simulink library "pixhawk_slib_rfly"  (R2022b)
settings: Solver=ode45  StartTime=0.0  StopTime=10.0  RelTol=1e-3
libraries: pixhawk_slib_uORB_RW x42, $bdroot x7
(part 2 of 3)

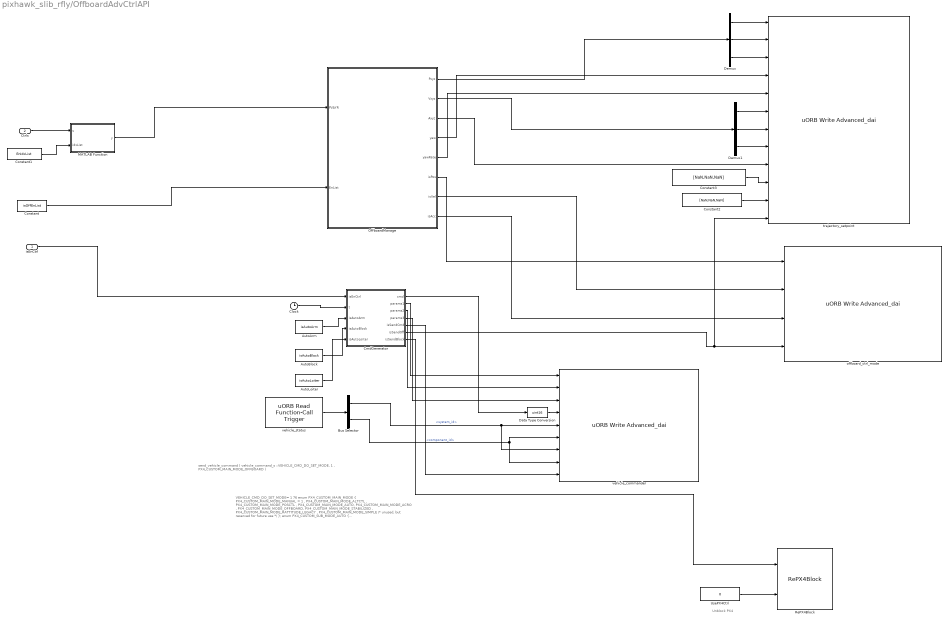
== system pixhawk_slib_rfly/OffboardAdvCtrlAPI ==
  note: VEHICLE_CMD_DO_SET_MODE= 1 76
      |
      | enum PX4_CUSTOM_MAIN_MODE {
      | PX4_CUSTOM_MAIN_MODE_MANUAL = 1 ,
      | PX4_CUSTOM_MAIN_MODE_ALTCTL ,
      | PX4_CUSTOM_MAIN_MODE_POSCTL ,
      | PX4_CUSTOM_MAIN_MODE_AUTO,
      | PX4_CUSTOM_MAIN_MODE_ACRO ,
      | PX4_CUSTOM_MAIN_MODE_OFFBOARD,
      | PX4_CUSTOM_MAIN_MODE_STABILIZED ,
      | PX4_CUSTOM_MAIN_MODE_RATTITUDE_LEGACY ,
      | PX4_CUSTOM_MAIN_MODE_SIMPLE /* unused, but reserved for future use */
      | };
      |
      | enum PX4_CUSTOM_SUB_MODE_AUTO {
      | PX4_CUSTOM_SUB_MODE_AUTO_READY = 1 ,
      | PX4_CUSTOM_SUB_MODE_AUTO_TAKEOFF ,
      | PX4_CUSTOM_SUB_MODE_AUTO_LOITER,
      | PX4_CUSTOM_SUB_MODE_AUTO_MISSION ,
      | PX4_CUSTOM_SUB_MODE_AUTO_RTL ,
      | PX4_CUSTOM_SUB_MODE_AUTO_LAND ,
      | PX4_CUSTOM_SUB_MODE_AUTO_RESERVED_DO_NOT_USE , // was PX4_CUSTOM_SUB_MODE_AUTO_RTGS, deleted 2020-03-05
      | PX4_CUSTOM_SUB_MODE_AUTO_FOLLOW_TARGET ,
      | PX4_CUSTOM_SUB_MODE_AUTO_PRECLAND
      | };
  note: Unblock PX4
  note: send_vehicle_command ( vehicle_command_s ::VEHICLE_CMD_DO_SET_MODE, 1 , PX4_CUSTOM_MAIN_MODE_OFFBOARD )
  isEnCtrl : Inport  OutDataTypeStr=boolean  PortDimensions=1
  Ctrls : Inport  Port=2  OutDataTypeStr=single  PortDimensions=4
  AutoArm : Constant  Value=isAutoArm  OutDataTypeStr=boolean
  AutoBlock : Constant  Value=isAutoBlock  OutDataTypeStr=boolean
  AutoLoiter : Constant  Value=isAutoLoiter  OutDataTypeStr=boolean
  Bus Selector : BusSelector  OutputSignals=system_id,component_id
  Clock : Clock
  CmdGenerator : MATLAB Function  TreatAsAtomicUnit=on  SystemSampleTime=SamTime
  Constant : Constant  Value=isOffEnList  OutDataTypeStr=boolean
  Constant1 : Constant  Value=EnIdxList
  Constant2 : Constant  Value=[NaN,NaN,NaN]  OutDataTypeStr=single
  Constant3 : Constant  Value=[NaN,NaN,NaN]  OutDataTypeStr=single
  Data Type Conversion : DataTypeConversion  OutDataTypeStr=uint16  SaturateOnIntegerOverflow=off  RndMeth=Floor
  Demux : Demux  Outputs=3
  Demux1 : Demux  Outputs=3
  MATLAB Function : MATLAB Function  TreatAsAtomicUnit=on  SystemSampleTime=SamTime
  OffboardManage : MATLAB Function  TreatAsAtomicUnit=on  SystemSampleTime=SamTime
  RePX4Block : $bdroot/RePX4Block  SamTime=SamTime
  UsePX4Ctrl : Constant  Value=0  OutDataTypeStr=uint8
  offboard_ctrl_mode : pixhawk_slib_uORB_RW/uORB Write Advanced_dai  Ts=0  uORB_AdvtQueue=on  uORB_FieldEnabledArr="0  0  0  1  0  0  0  0  0  0  0"  uORB_Topic_str=0  uORB_Topic_str_ID=0  uORB_Struct_DT="[1  1  1  1  1]"  BlockInputCount=5  uORB_StructParams="[\"voltage_v\",\"voltage_filtered_v\",\"current_a\",\"current_filtered_a\",\"remaining\"]"  uORB_PortSizes="[1  1  1  1]"  MsgSizeOf=0  MW_update=true
      settings: SourceProductName=Pixhawk Target Blocks
  trajectory_setpoint : pixhawk_slib_uORB_RW/uORB Write Advanced_dai  Ts=0  uORB_AdvtQueue=on  uORB_FieldEnabledArr="0  0  0  1  0  0  0  0  0  0  0"  uORB_Topic_str=0  uORB_Topic_str_ID=0  uORB_Struct_DT="[1  1  1  1  1]"  BlockInputCount=5  uORB_StructParams="[\"voltage_v\",\"voltage_filtered_v\",\"current_a\",\"current_filtered_a\",\"remaining\"]"  uORB_PortSizes="[1  1  1  1]"  MsgSizeOf=0  MW_update=true
      settings: SourceProductName=Pixhawk Target Blocks
  vehicle_commander : pixhawk_slib_uORB_RW/uORB Write Advanced_dai  Ts=0  uORB_AdvtQueue=on  uORB_FieldEnabledArr="0  0  0  1  0  0  0  0  0  0  0"  uORB_Topic_str=0  uORB_Topic_str_ID=0  uORB_Struct_DT="[1  1  1  1  1]"  BlockInputCount=5  uORB_StructParams="[\"voltage_v\",\"voltage_filtered_v\",\"current_a\",\"current_filtered_a\",\"remaining\"]"  uORB_PortSizes="[1  1  1  1]"  MsgSizeOf=0  MW_update=true
      settings: SourceProductName=Pixhawk Target Blocks
  vehicle_status : pixhawk_slib_uORB_RW/uORB Read Function-Call Trigger  uORB_Topic_str='vehicle_status'  BusObjVar=Bus: vehicle_status_SL  uORB_Interval=50  AsyncOutput=off  Fcn_call_select=Generate Function Call Signal  TaskName='Task1'  Poll_timeout=-1  Ts=SamTime
      settings: SourceProductName=Pixhawk Target Blocks
  wires:
  Ctrls/1 -> MATLAB Function/1(u)
  Constant1/1 -> MATLAB Function/2(idxList)
  Bus Selector/2 -> vehicle_commander/8, vehicle_commander/6  "<component_id>"
  CmdGenerator/5(isSendCmd) -> vehicle_commander/9
  Clock/1 -> CmdGenerator/2(t)
  OffboardManage/6(isPos) -> offboard_ctrl_mode/1
  OffboardManage/7(isVel) -> offboard_ctrl_mode/2
  AutoLoiter/1 -> CmdGenerator/5(isAutoLoiter)
  UsePX4Ctrl/1 -> RePX4Block/2
  AutoBlock/1 -> CmdGenerator/4(isAutoBlock)
  Constant/1 -> OffboardManage/2(EnList)
  CmdGenerator/4(params3) -> vehicle_commander/3
  CmdGenerator/1(cmd) -> Data Type Conversion/1
  CmdGenerator/3(params2) -> vehicle_commander/2
  AutoArm/1 -> CmdGenerator/3(isAutoArm)
  OffboardManage/8(isAcc) -> offboard_ctrl_mode/3
  CmdGenerator/2(params1) -> vehicle_commander/1
  CmdGenerator/7(isSendBlock) -> RePX4Block/1
  vehicle_status/1 -> Bus Selector/1
  MATLAB Function/1(y) -> OffboardManage/1(PVAYR)
  Bus Selector/1 -> vehicle_commander/7, vehicle_commander/5  "<system_id>"
  isEnCtrl/1 -> CmdGenerator/1(isEnCtrl)
  Demux1/3 -> trajectory_setpoint/8
  Demux1/1 -> trajectory_setpoint/6
  Demux/3 -> trajectory_setpoint/3
  Demux1/2 -> trajectory_setpoint/7
  Demux/1 -> trajectory_setpoint/1
  Demux/2 -> trajectory_setpoint/2
  OffboardManage/5(yawRate) -> trajectory_setpoint/5
  OffboardManage/3(Axyz) -> trajectory_setpoint/9
  Constant2/1 -> trajectory_setpoint/11
  OffboardManage/4(yaw) -> trajectory_setpoint/4
  Constant3/1 -> trajectory_setpoint/10
  OffboardManage/1(Pxyz) -> Demux/1
  CmdGenerator/6(isSendOff) -> trajectory_setpoint/12, offboard_ctrl_mode/4
  OffboardManage/2(Vxyz) -> Demux1/1
  Data Type Conversion/1 -> vehicle_commander/4

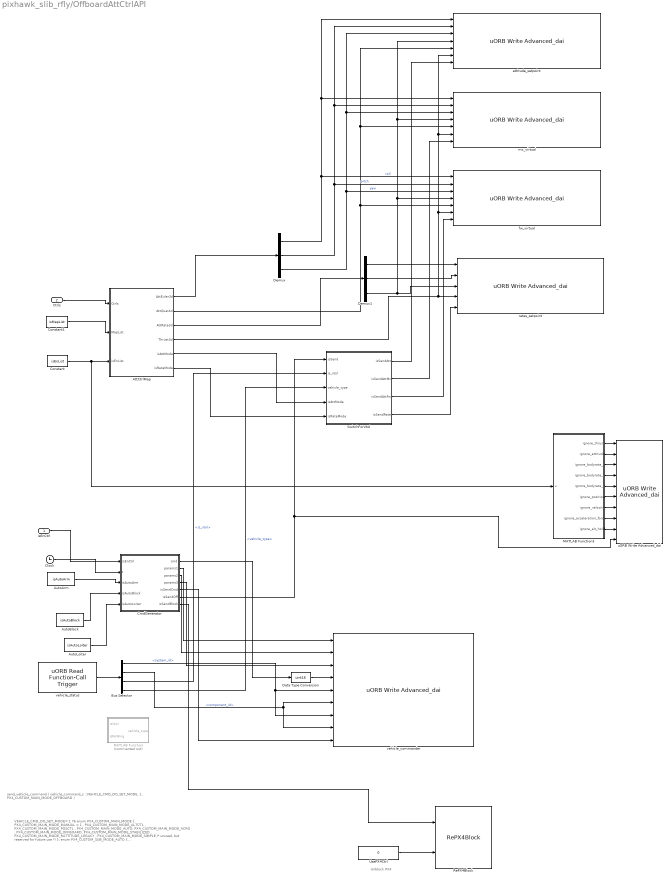
== system pixhawk_slib_rfly/OffboardAttCtrlAPI ==
  note: Unblock PX4
  note: VEHICLE_CMD_DO_SET_MODE= 1 76
      |
      | enum PX4_CUSTOM_MAIN_MODE {
      | PX4_CUSTOM_MAIN_MODE_MANUAL = 1 ,
      | PX4_CUSTOM_MAIN_MODE_ALTCTL ,
      | PX4_CUSTOM_MAIN_MODE_POSCTL ,
      | PX4_CUSTOM_MAIN_MODE_AUTO,
      | PX4_CUSTOM_MAIN_MODE_ACRO ,
      | PX4_CUSTOM_MAIN_MODE_OFFBOARD,
      | PX4_CUSTOM_MAIN_MODE_STABILIZED ,
      | PX4_CUSTOM_MAIN_MODE_RATTITUDE_LEGACY ,
      | PX4_CUSTOM_MAIN_MODE_SIMPLE /* unused, but reserved for future use */
      | };
      |
      | enum PX4_CUSTOM_SUB_MODE_AUTO {
      | PX4_CUSTOM_SUB_MODE_AUTO_READY = 1 ,
      | PX4_CUSTOM_SUB_MODE_AUTO_TAKEOFF ,
      | PX4_CUSTOM_SUB_MODE_AUTO_LOITER,
      | PX4_CUSTOM_SUB_MODE_AUTO_MISSION ,
      | PX4_CUSTOM_SUB_MODE_AUTO_RTL ,
      | PX4_CUSTOM_SUB_MODE_AUTO_LAND ,
      | PX4_CUSTOM_SUB_MODE_AUTO_RESERVED_DO_NOT_USE , // was PX4_CUSTOM_SUB_MODE_AUTO_RTGS, deleted 2020-03-05
      | PX4_CUSTOM_SUB_MODE_AUTO_FOLLOW_TARGET ,
      | PX4_CUSTOM_SUB_MODE_AUTO_PRECLAND
      | };
  note: send_vehicle_command ( vehicle_command_s ::VEHICLE_CMD_DO_SET_MODE, 1 , PX4_CUSTOM_MAIN_MODE_OFFBOARD )
  isEnCtrl : Inport  OutDataTypeStr=boolean  PortDimensions=1
  Ctrls : Inport  Port=2  OutDataTypeStr=single  PortDimensions=6
  AttCtrlMap : MATLAB Function  TreatAsAtomicUnit=on  SystemSampleTime=SamTime
  AutoArm : Constant  Value=isAutoArm  OutDataTypeStr=boolean
  AutoBlock : Constant  Value=isAutoBlock  OutDataTypeStr=boolean
  AutoLoiter : Constant  Value=isAutoLoiter  OutDataTypeStr=boolean
  Bus Selector : BusSelector  OutputSignals=system_id,component_id,is_vtol,vehicle_type
  Clock : Clock
  CmdGenerator : MATLAB Function  TreatAsAtomicUnit=on  SystemSampleTime=SamTime
  Constant : Constant  Value=isEnList  OutDataTypeStr=boolean
  Constant1 : Constant  Value=isMapList
  Data Type Conversion : DataTypeConversion  OutDataTypeStr=uint16  SaturateOnIntegerOverflow=off  RndMeth=Floor
  Demux : Demux  Outputs=3
  Demux1 : Demux  Outputs=3
  MATLAB Function : MATLAB Function  Commented=on  TreatAsAtomicUnit=on
  MATLAB Function3 : MATLAB Function  TreatAsAtomicUnit=on
  RePX4Block : $bdroot/RePX4Block  SamTime=SamTime
  SwitchForVtol : MATLAB Function  TreatAsAtomicUnit=on  SystemSampleTime=SamTime
  UsePX4Ctrl : Constant  Value=0  OutDataTypeStr=uint8
  attitude_setpoint : pixhawk_slib_uORB_RW/uORB Write Advanced_dai  Ts=0  uORB_AdvtQueue=on  uORB_FieldEnabledArr="0  0  0  1  0  0  0  0  0  0  0"  uORB_Topic_str=0  uORB_Topic_str_ID=0  uORB_Struct_DT="[1  1  1  1  1]"  BlockInputCount=5  uORB_StructParams="[\"voltage_v\",\"voltage_filtered_v\",\"current_a\",\"current_filtered_a\",\"remaining\"]"  uORB_PortSizes="[1  1  1  1]"  MsgSizeOf=0  MW_update=true
      settings: SourceProductName=Pixhawk Target Blocks
  fw_virtual : pixhawk_slib_uORB_RW/uORB Write Advanced_dai  Ts=0  uORB_AdvtQueue=on  uORB_FieldEnabledArr="0  0  0  1  0  0  0  0  0  0  0"  uORB_Topic_str=0  uORB_Topic_str_ID=0  uORB_Struct_DT="[1  1  1  1  1]"  BlockInputCount=5  uORB_StructParams="[\"voltage_v\",\"voltage_filtered_v\",\"current_a\",\"current_filtered_a\",\"remaining\"]"  uORB_PortSizes="[1  1  1  1]"  MsgSizeOf=0  MW_update=true
      settings: SourceProductName=Pixhawk Target Blocks
  mc_virtual : pixhawk_slib_uORB_RW/uORB Write Advanced_dai  Ts=0  uORB_AdvtQueue=on  uORB_FieldEnabledArr="0  0  0  1  0  0  0  0  0  0  0"  uORB_Topic_str=0  uORB_Topic_str_ID=0  uORB_Struct_DT="[1  1  1  1  1]"  BlockInputCount=5  uORB_StructParams="[\"voltage_v\",\"voltage_filtered_v\",\"current_a\",\"current_filtered_a\",\"remaining\"]"  uORB_PortSizes="[1  1  1  1]"  MsgSizeOf=0  MW_update=true
      settings: SourceProductName=Pixhawk Target Blocks
  rates_setpoint : pixhawk_slib_uORB_RW/uORB Write Advanced_dai  Ts=0  uORB_AdvtQueue=on  uORB_FieldEnabledArr="0  0  0  1  0  0  0  0  0  0  0"  uORB_Topic_str=0  uORB_Topic_str_ID=0  uORB_Struct_DT="[1  1  1  1  1]"  BlockInputCount=5  uORB_StructParams="[\"voltage_v\",\"voltage_filtered_v\",\"current_a\",\"current_filtered_a\",\"remaining\"]"  uORB_PortSizes="[1  1  1  1]"  MsgSizeOf=0  MW_update=true
      settings: SourceProductName=Pixhawk Target Blocks
  uORB Write Advanced_dai : pixhawk_slib_uORB_RW/uORB Write Advanced_dai  Ts=0  uORB_AdvtQueue=on  uORB_FieldEnabledArr="0  0  0  1  0  0  0  0  0  0  0"  uORB_Topic_str=0  uORB_Topic_str_ID=0  uORB_Struct_DT="[1  1  1  1  1]"  BlockInputCount=5  uORB_StructParams="[\"voltage_v\",\"voltage_filtered_v\",\"current_a\",\"current_filtered_a\",\"remaining\"]"  uORB_PortSizes="[1  1  1  1]"  MsgSizeOf=0  MW_update=true
      settings: SourceProductName=Pixhawk Target Blocks
  vehicle_commander : pixhawk_slib_uORB_RW/uORB Write Advanced_dai  Ts=0  uORB_AdvtQueue=on  uORB_FieldEnabledArr="0  0  0  1  0  0  0  0  0  0  0"  uORB_Topic_str=0  uORB_Topic_str_ID=0  uORB_Struct_DT="[1  1  1  1  1]"  BlockInputCount=5  uORB_StructParams="[\"voltage_v\",\"voltage_filtered_v\",\"current_a\",\"current_filtered_a\",\"remaining\"]"  uORB_PortSizes="[1  1  1  1]"  MsgSizeOf=0  MW_update=true
      settings: SourceProductName=Pixhawk Target Blocks
  vehicle_status : pixhawk_slib_uORB_RW/uORB Read Function-Call Trigger  uORB_Topic_str='vehicle_status'  BusObjVar=Bus: vehicle_status_SL  uORB_Interval=50  AsyncOutput=off  Fcn_call_select=Generate Function Call Signal  TaskName='Task1'  Poll_timeout=-1  Ts=SamTime
      settings: SourceProductName=Pixhawk Target Blocks
  wires:
  AttCtrlMap/5(isAttMode) -> SwitchForVtol/4(isAttMode)
  AttCtrlMap/6(isRateMode) -> SwitchForVtol/5(isRateMode)
  Constant1/1 -> AttCtrlMap/2(MapList)
  Constant/1 -> MATLAB Function3/1(u), AttCtrlMap/3(isEnList)
  AttCtrlMap/1(AttEuler3d) -> Demux/1
  Demux/1 -> attitude_setpoint/1, mc_virtual/1, fw_virtual/1  "roll"
  Demux/2 -> fw_virtual/2, mc_virtual/2, attitude_setpoint/2  "pitch"
  Demux/3 -> fw_virtual/3, mc_virtual/3, attitude_setpoint/3  "yaw"
  AttCtrlMap/3(AttRate3d) -> Demux1/1
  Demux1/1 -> rates_setpoint/1
  Demux1/2 -> rates_setpoint/2
  Demux1/3 -> fw_virtual/4, mc_virtual/4, attitude_setpoint/4, rates_setpoint/3
  AttCtrlMap/2(AttQuat4d) -> fw_virtual/5, mc_virtual/5, attitude_setpoint/5
  AttCtrlMap/4(Thrust3d) -> attitude_setpoint/6, mc_virtual/6, fw_virtual/6, rates_setpoint/4
  SwitchForVtol/1(isSendAtt) -> attitude_setpoint/7
  SwitchForVtol/2(isSendAttMc) -> mc_virtual/7
  SwitchForVtol/3(isSendAttFw) -> fw_virtual/7
  SwitchForVtol/4(isSendRate) -> rates_setpoint/5
  Ctrls/1 -> AttCtrlMap/1(Ctrls)
  AutoLoiter/1 -> CmdGenerator/5(isAutoLoiter)
  CmdGenerator/4(params3) -> vehicle_commander/3
  CmdGenerator/3(params2) -> vehicle_commander/2
  CmdGenerator/7(isSendBlock) -> RePX4Block/1
  AutoBlock/1 -> CmdGenerator/4(isAutoBlock)
  AutoArm/1 -> CmdGenerator/3(isAutoArm)
  CmdGenerator/1(cmd) -> Data Type Conversion/1
  UsePX4Ctrl/1 -> RePX4Block/2
  Clock/1 -> CmdGenerator/2(t)
  CmdGenerator/2(params1) -> vehicle_commander/1
  CmdGenerator/5(isSendCmd) -> vehicle_commander/9
  Bus Selector/1 -> vehicle_commander/7, vehicle_commander/5  "<system_id>"
  isEnCtrl/1 -> CmdGenerator/1(isEnCtrl)
  CmdGenerator/6(isSendOff) -> SwitchForVtol/1(isSend), uORB Write Advanced_dai/10
  Bus Selector/2 -> vehicle_commander/8, vehicle_commander/6  "<component_id>"
  vehicle_status/1 -> Bus Selector/1
  Bus Selector/3 -> SwitchForVtol/2(is_vtol)  "<is_vtol>"
  Bus Selector/4 -> SwitchForVtol/3(vehicle_type)  "<vehicle_type>"
  MATLAB Function3/1(ignore_thrust) -> uORB Write Advanced_dai/1
  MATLAB Function3/2(ignore_attitude) -> uORB Write Advanced_dai/2
  MATLAB Function3/3(ignore_bodyrate_x) -> uORB Write Advanced_dai/3
  MATLAB Function3/4(ignore_bodyrate_y) -> uORB Write Advanced_dai/4
  MATLAB Function3/5(ignore_bodyrate_z) -> uORB Write Advanced_dai/5
  MATLAB Function3/6(ignore_position) -> uORB Write Advanced_dai/6
  MATLAB Function3/7(ignore_velocity) -> uORB Write Advanced_dai/7
  MATLAB Function3/8(ignore_acceleration_force) -> uORB Write Advanced_dai/8
  MATLAB Function3/9(ignore_alt_hold) -> uORB Write Advanced_dai/9
  Data Type Conversion/1 -> vehicle_commander/4

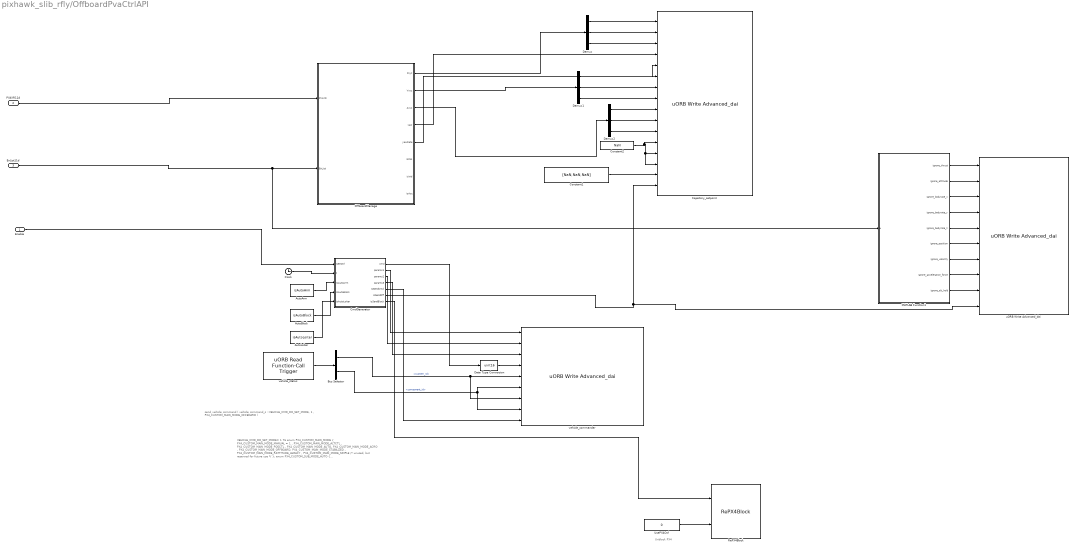
== system pixhawk_slib_rfly/OffboardPvaCtrlAPI ==
  note: Unblock PX4
  note: VEHICLE_CMD_DO_SET_MODE= 1 76
      |
      | enum PX4_CUSTOM_MAIN_MODE {
      | PX4_CUSTOM_MAIN_MODE_MANUAL = 1 ,
      | PX4_CUSTOM_MAIN_MODE_ALTCTL ,
      | PX4_CUSTOM_MAIN_MODE_POSCTL ,
      | PX4_CUSTOM_MAIN_MODE_AUTO,
      | PX4_CUSTOM_MAIN_MODE_ACRO ,
      | PX4_CUSTOM_MAIN_MODE_OFFBOARD,
      | PX4_CUSTOM_MAIN_MODE_STABILIZED ,
      | PX4_CUSTOM_MAIN_MODE_RATTITUDE_LEGACY ,
      | PX4_CUSTOM_MAIN_MODE_SIMPLE /* unused, but reserved for future use */
      | };
      |
      | enum PX4_CUSTOM_SUB_MODE_AUTO {
      | PX4_CUSTOM_SUB_MODE_AUTO_READY = 1 ,
      | PX4_CUSTOM_SUB_MODE_AUTO_TAKEOFF ,
      | PX4_CUSTOM_SUB_MODE_AUTO_LOITER,
      | PX4_CUSTOM_SUB_MODE_AUTO_MISSION ,
      | PX4_CUSTOM_SUB_MODE_AUTO_RTL ,
      | PX4_CUSTOM_SUB_MODE_AUTO_LAND ,
      | PX4_CUSTOM_SUB_MODE_AUTO_RESERVED_DO_NOT_USE , // was PX4_CUSTOM_SUB_MODE_AUTO_RTGS, deleted 2020-03-05
      | PX4_CUSTOM_SUB_MODE_AUTO_FOLLOW_TARGET ,
      | PX4_CUSTOM_SUB_MODE_AUTO_PRECLAND
      | };
  note: send_vehicle_command ( vehicle_command_s ::VEHICLE_CMD_DO_SET_MODE, 1 , PX4_CUSTOM_MAIN_MODE_OFFBOARD )
  Enable : Inport  OutDataTypeStr=boolean  PortDimensions=1
  PVAYR11d : Inport  Port=2  OutDataTypeStr=single  PortDimensions=11
  EnList11d : Inport  Port=3  OutDataTypeStr=boolean  PortDimensions=11
  AutoArm : Constant  Value=isAutoArm  OutDataTypeStr=boolean
  AutoBlock : Constant  Value=isAutoBlock  OutDataTypeStr=boolean
  AutoLoiter : Constant  Value=isAutoLoiter  OutDataTypeStr=boolean
  Bus Selector : BusSelector  OutputSignals=system_id,component_id
  Clock : Clock
  CmdGenerator : MATLAB Function  TreatAsAtomicUnit=on  SystemSampleTime=SamTime
  Constant1 : Constant  Value=[NaN,NaN,NaN]  OutDataTypeStr=single
  Constant2 : Constant  Value=NaN  OutDataTypeStr=single
  Data Type Conversion : DataTypeConversion  OutDataTypeStr=uint16  SaturateOnIntegerOverflow=off  RndMeth=Floor
  Demux : Demux  Outputs=3
  Demux1 : Demux  Outputs=3
  Demux2 : Demux  Outputs=3
  MATLAB Function1 : MATLAB Function  TreatAsAtomicUnit=on
  OffboardManage : MATLAB Function  TreatAsAtomicUnit=on  SystemSampleTime=SamTime
  RePX4Block : $bdroot/RePX4Block  SamTime=SamTime
  UsePX4Ctrl : Constant  Value=0  OutDataTypeStr=uint8
  trajectory_setpoint : pixhawk_slib_uORB_RW/uORB Write Advanced_dai  Ts=0  uORB_AdvtQueue=on  uORB_FieldEnabledArr="0  0  0  1  0  0  0  0  0  0  0"  uORB_Topic_str=0  uORB_Topic_str_ID=0  uORB_Struct_DT="[1  1  1  1  1]"  BlockInputCount=5  uORB_StructParams="[\"voltage_v\",\"voltage_filtered_v\",\"current_a\",\"current_filtered_a\",\"remaining\"]"  uORB_PortSizes="[1  1  1  1]"  MsgSizeOf=0  MW_update=true
      settings: SourceProductName=Pixhawk Target Blocks
  uORB Write Advanced_dai : pixhawk_slib_uORB_RW/uORB Write Advanced_dai  Ts=0  uORB_AdvtQueue=on  uORB_FieldEnabledArr="0  0  0  1  0  0  0  0  0  0  0"  uORB_Topic_str=0  uORB_Topic_str_ID=0  uORB_Struct_DT="[1  1  1  1  1]"  BlockInputCount=5  uORB_StructParams="[\"voltage_v\",\"voltage_filtered_v\",\"current_a\",\"current_filtered_a\",\"remaining\"]"  uORB_PortSizes="[1  1  1  1]"  MsgSizeOf=0  MW_update=true
      settings: SourceProductName=Pixhawk Target Blocks
  vehicle_commander : pixhawk_slib_uORB_RW/uORB Write Advanced_dai  Ts=0  uORB_AdvtQueue=on  uORB_FieldEnabledArr="0  0  0  1  0  0  0  0  0  0  0"  uORB_Topic_str=0  uORB_Topic_str_ID=0  uORB_Struct_DT="[1  1  1  1  1]"  BlockInputCount=5  uORB_StructParams="[\"voltage_v\",\"voltage_filtered_v\",\"current_a\",\"current_filtered_a\",\"remaining\"]"  uORB_PortSizes="[1  1  1  1]"  MsgSizeOf=0  MW_update=true
      settings: SourceProductName=Pixhawk Target Blocks
  vehicle_status : pixhawk_slib_uORB_RW/uORB Read Function-Call Trigger  uORB_Topic_str='vehicle_status'  BusObjVar=Bus: vehicle_status_SL  uORB_Interval=50  AsyncOutput=off  Fcn_call_select=Generate Function Call Signal  TaskName='Task1'  Poll_timeout=-1  Ts=SamTime
      settings: SourceProductName=Pixhawk Target Blocks
  wires:
  Enable/1 -> CmdGenerator/1(isEnCtrl)
  vehicle_status/1 -> Bus Selector/1
  CmdGenerator/1(cmd) -> Data Type Conversion/1
  Clock/1 -> CmdGenerator/2(t)
  EnList11d/1 -> MATLAB Function1/1(u), OffboardManage/2(EnList)
  CmdGenerator/5(isSendCmd) -> vehicle_commander/9
  Bus Selector/1 -> vehicle_commander/7, vehicle_commander/5  "<system_id>"
  Bus Selector/2 -> vehicle_commander/8, vehicle_commander/6  "<component_id>"
  AutoArm/1 -> CmdGenerator/3(isAutoArm)
  AutoBlock/1 -> CmdGenerator/4(isAutoBlock)
  CmdGenerator/7(isSendBlock) -> RePX4Block/1
  UsePX4Ctrl/1 -> RePX4Block/2
  CmdGenerator/2(params1) -> vehicle_commander/1
  CmdGenerator/3(params2) -> vehicle_commander/2
  CmdGenerator/4(params3) -> vehicle_commander/3
  AutoLoiter/1 -> CmdGenerator/5(isAutoLoiter)
  PVAYR11d/1 -> OffboardManage/1(PVAYR)
  CmdGenerator/6(isSendOff) -> uORB Write Advanced_dai/10, trajectory_setpoint/16
  Demux/2 -> trajectory_setpoint/2
  Demux/1 -> trajectory_setpoint/1
  Demux1/1 -> trajectory_setpoint/6
  Demux/3 -> trajectory_setpoint/3
  Demux1/2 -> trajectory_setpoint/7
  Constant1/1 -> trajectory_setpoint/15
  Demux1/3 -> trajectory_setpoint/8
  OffboardManage/1(Pxyz) -> Demux/1
  OffboardManage/2(Vxyz) -> Demux1/1
  OffboardManage/3(Axyz) -> Demux2/1
  OffboardManage/4(yaw) -> trajectory_setpoint/4
  OffboardManage/5(yawRate) -> trajectory_setpoint/5
  Demux2/1 -> trajectory_setpoint/9
  Demux2/2 -> trajectory_setpoint/10
  Demux2/3 -> trajectory_setpoint/11
  Constant2/1 -> trajectory_setpoint/14, trajectory_setpoint/13, trajectory_setpoint/12
  MATLAB Function1/1(ignore_thrust) -> uORB Write Advanced_dai/1
  MATLAB Function1/2(ignore_attitude) -> uORB Write Advanced_dai/2
  MATLAB Function1/3(ignore_bodyrate_x) -> uORB Write Advanced_dai/3
  MATLAB Function1/4(ignore_bodyrate_y) -> uORB Write Advanced_dai/4
  MATLAB Function1/5(ignore_bodyrate_z) -> uORB Write Advanced_dai/5
  MATLAB Function1/6(ignore_position) -> uORB Write Advanced_dai/6
  MATLAB Function1/7(ignore_velocity) -> uORB Write Advanced_dai/7
  MATLAB Function1/8(ignore_acceleration_force) -> uORB Write Advanced_dai/8
  MATLAB Function1/9(ignore_alt_hold) -> uORB Write Advanced_dai/9
  Data Type Conversion/1 -> vehicle_commander/4

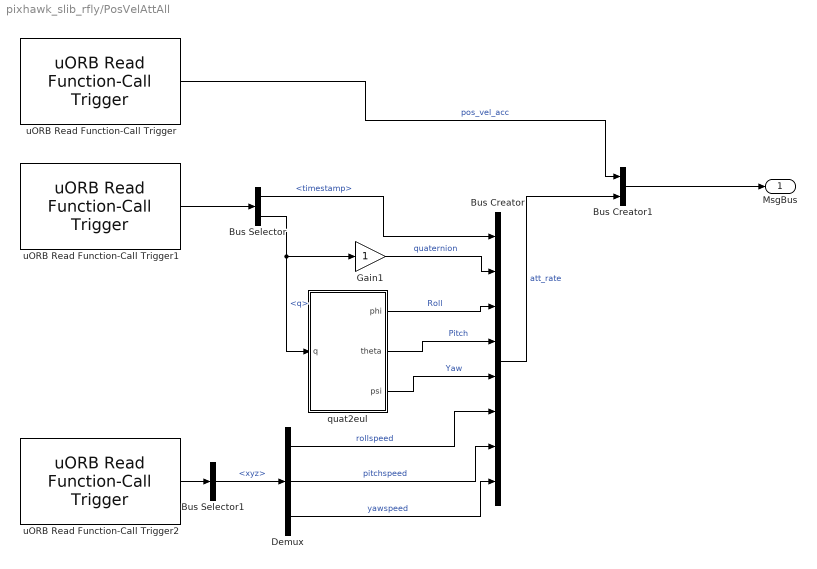
== system pixhawk_slib_rfly/PosVelAttAll ==
  Bus Creator : BusCreator  Inputs=8
  Bus Creator1 : BusCreator  Inputs=2
  Bus Selector : BusSelector  OutputSignals=timestamp,q
  Bus Selector1 : BusSelector  OutputSignals=xyz
  Demux : Demux  Outputs=3
  Gain1 : Gain
  quat2eul : MATLAB Function  TreatAsAtomicUnit=on
  uORB Read Function-Call Trigger : pixhawk_slib_uORB_RW/uORB Read Function-Call Trigger  uORB_Topic_str='vehicle_local_position'  BusObjVar=Bus: vehicle_local_position_SL  uORB_Interval=4  AsyncOutput=off  Fcn_call_select=Generate Function Call Signal  TaskName='Task1'  Poll_timeout=-1  Ts=SamTime
      settings: SourceProductName=Pixhawk Target Blocks
  uORB Read Function-Call Trigger1 : pixhawk_slib_uORB_RW/uORB Read Function-Call Trigger  uORB_Topic_str='vehicle_attitude'  BusObjVar=Bus: vehicle_attitude_SL  uORB_Interval=4  AsyncOutput=off  Fcn_call_select=Generate Function Call Signal  TaskName='Task1'  Poll_timeout=-1  Ts=SamTime
      settings: SourceProductName=Pixhawk Target Blocks
  uORB Read Function-Call Trigger2 : pixhawk_slib_uORB_RW/uORB Read Function-Call Trigger  uORB_Topic_str='vehicle_angular_velocity'  BusObjVar=Bus: vehicle_angular_velocity_SL  uORB_Interval=4  AsyncOutput=off  Fcn_call_select=Generate Function Call Signal  TaskName='Task1'  Poll_timeout=-1  Ts=SamTime
      settings: SourceProductName=Pixhawk Target Blocks
  MsgBus : Outport  VectorParamsAs1DForOutWhenUnconnected=off
  wires:
  Bus Creator1/1 -> MsgBus/1
  Bus Selector/1 -> Bus Creator/1  "<timestamp>"
  Bus Selector1/1 -> Demux/1  "<xyz>"
  Gain1/1 -> Bus Creator/2  "quaternion"
  Bus Selector/2 -> quat2eul/1(q), Gain1/1  "<q>"
  uORB Read Function-Call Trigger2/1 -> Bus Selector1/1
  quat2eul/1(phi) -> Bus Creator/3  "Roll"
  Demux/1 -> Bus Creator/6  "rollspeed"
  Demux/3 -> Bus Creator/8  "yawspeed"
  quat2eul/3(psi) -> Bus Creator/5  "Yaw"
  Demux/2 -> Bus Creator/7  "pitchspeed"
  quat2eul/2(theta) -> Bus Creator/4  "Pitch"
  uORB Read Function-Call Trigger/1 -> Bus Creator1/1  "pos_vel_acc"
  Bus Creator/1 -> Bus Creator1/2  "att_rate"
  uORB Read Function-Call Trigger1/1 -> Bus Selector/1

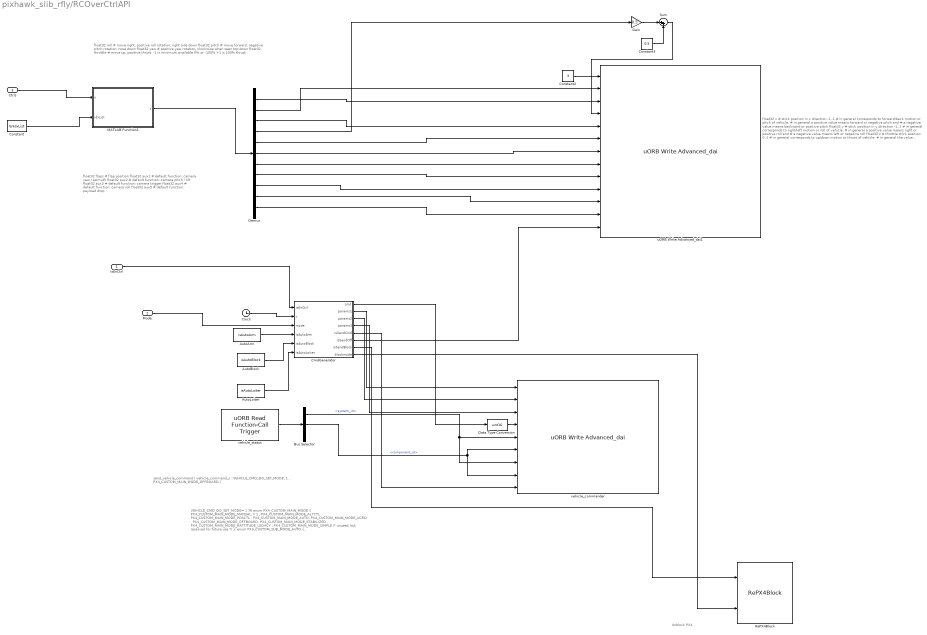
== system pixhawk_slib_rfly/RCOverCtrlAPI ==
  note: send_vehicle_command ( vehicle_command_s ::VEHICLE_CMD_DO_SET_MODE, 1 , PX4_CUSTOM_MAIN_MODE_OFFBOARD )
  note: Unblock PX4
  note: VEHICLE_CMD_DO_SET_MODE= 1 76
      |
      | enum PX4_CUSTOM_MAIN_MODE {
      | PX4_CUSTOM_MAIN_MODE_MANUAL = 1 ,
      | PX4_CUSTOM_MAIN_MODE_ALTCTL ,
      | PX4_CUSTOM_MAIN_MODE_POSCTL ,
      | PX4_CUSTOM_MAIN_MODE_AUTO,
      | PX4_CUSTOM_MAIN_MODE_ACRO ,
      | PX4_CUSTOM_MAIN_MODE_OFFBOARD,
      | PX4_CUSTOM_MAIN_MODE_STABILIZED ,
      | PX4_CUSTOM_MAIN_MODE_RATTITUDE_LEGACY ,
      | PX4_CUSTOM_MAIN_MODE_SIMPLE /* unused, but reserved for future use */
      | };
      |
      | enum PX4_CUSTOM_SUB_MODE_AUTO {
      | PX4_CUSTOM_SUB_MODE_AUTO_READY = 1 ,
      | PX4_CUSTOM_SUB_MODE_AUTO_TAKEOFF ,
      | PX4_CUSTOM_SUB_MODE_AUTO_LOITER,
      | PX4_CUSTOM_SUB_MODE_AUTO_MISSION ,
      | PX4_CUSTOM_SUB_MODE_AUTO_RTL ,
      | PX4_CUSTOM_SUB_MODE_AUTO_LAND ,
      | PX4_CUSTOM_SUB_MODE_AUTO_RESERVED_DO_NOT_USE , // was PX4_CUSTOM_SUB_MODE_AUTO_RTGS, deleted 2020-03-05
      | PX4_CUSTOM_SUB_MODE_AUTO_FOLLOW_TARGET ,
      | PX4_CUSTOM_SUB_MODE_AUTO_PRECLAND
      | };
  note: float32 flaps			 # flap position
      |
      | float32 aux1			 # default function: camera yaw / azimuth
      | float32 aux2			 # default function: camera pitch / tilt
      | float32 aux3			 # default function: camera trigger
      | float32 aux4			 # default function: camera roll
      | float32 aux5			 # default function: payload drop
  note: float32 roll     # move right,   positive roll rotation,  right side down
      | float32 pitch    # move forward, negative pitch rotation, nose down
      | float32 yaw      #               positive yaw rotation,   clockwise when seen top down
      | float32 throttle # move up,      positive thrust,         -1 is minimum available 0% or -100% +1 is 100% thrust
  note: float32 x			 # stick position in x direction -1..1
      | 				 # in general corresponds to forward/back motion or pitch of vehicle,
      | 				 # in general a positive value means forward or negative pitch and
      | 				 # a negative value means backward or positive pitch
      |
      | float32 y			 # stick position in y direction -1..1
      | 				 # in general corresponds to right/left motion or roll of vehicle,
      | 				 # in general a positive value means right or positive roll and
      | 				 # a negative value means left or negative roll
      |
      | float32 z			 # throttle stick position 0..1
      | 				 # in general corresponds to up/down motion or thrust of vehicle,
      | 				 # in general the value corresponds to the demanded throttle by the user,
      | 				 # if the input is used for setting the setpoint of a vertical position
      | 				 # controller any value > 0.5 means up and any value < 0.5 means down
      |
      | float32 r			 # yaw stick/twist position, -1..1
      | 				 # in general corresponds to the righthand rotation around the vertical
      | 				 # (downwards) axis of the vehicle
  isEnCtrl : Inport  OutDataTypeStr=boolean  PortDimensions=1
  Mode : Inport  Port=2  OutDataTypeStr=uint8  PortDimensions=1
  Ctrls : Inport  Port=3  OutDataTypeStr=single  PortDimensions=4
  AutoArm : Constant  Value=isAutoArm  OutDataTypeStr=boolean
  AutoBlock : Constant  Value=isAutoBlock  OutDataTypeStr=boolean
  AutoLoiter : Constant  Value=isAutoLoiter  OutDataTypeStr=boolean
  Bus Selector : BusSelector  OutputSignals=system_id,component_id,timestamp
  Clock : Clock
  CmdGenerator : MATLAB Function  TreatAsAtomicUnit=on  SystemSampleTime=SamTime
  Constant : Constant  Value=EnIdxList
  Constant2 : Constant  Value=3  OutDataTypeStr=uint8
  Constant3 : Constant  Value=0.5  OutDataTypeStr=single
  Data Type Conversion : DataTypeConversion  OutDataTypeStr=uint16  SaturateOnIntegerOverflow=off  RndMeth=Floor
  Demux : Demux  Outputs=11
  Gain : Gain  Gain=0.5
  MATLAB Function1 : MATLAB Function  TreatAsAtomicUnit=on  SystemSampleTime=SamTime
  RePX4Block : $bdroot/RePX4Block  SamTime=SamTime
  Sum : Sum  Inputs=|++
  uORB Write Advanced_dai1 : pixhawk_slib_uORB_RW/uORB Write Advanced_dai  Ts=0  uORB_AdvtQueue=on  uORB_FieldEnabledArr="0  0  0  1  0  0  0  0  0  0  0"  uORB_Topic_str=0  uORB_Topic_str_ID=0  uORB_Struct_DT="[1  1  1  1  1]"  BlockInputCount=5  uORB_StructParams="[\"voltage_v\",\"voltage_filtered_v\",\"current_a\",\"current_filtered_a\",\"remaining\"]"  uORB_PortSizes="[1  1  1  1]"  MsgSizeOf=0  MW_update=true
      settings: SourceProductName=Pixhawk Target Blocks
  vehicle_commander : pixhawk_slib_uORB_RW/uORB Write Advanced_dai  Ts=0  uORB_AdvtQueue=on  uORB_FieldEnabledArr="0  0  0  1  0  0  0  0  0  0  0"  uORB_Topic_str=0  uORB_Topic_str_ID=0  uORB_Struct_DT="[1  1  1  1  1]"  BlockInputCount=5  uORB_StructParams="[\"voltage_v\",\"voltage_filtered_v\",\"current_a\",\"current_filtered_a\",\"remaining\"]"  uORB_PortSizes="[1  1  1  1]"  MsgSizeOf=0  MW_update=true
      settings: SourceProductName=Pixhawk Target Blocks
  vehicle_status : pixhawk_slib_uORB_RW/uORB Read Function-Call Trigger  uORB_Topic_str='vehicle_status'  BusObjVar=Bus: vehicle_status_SL  uORB_Interval=50  AsyncOutput=off  Fcn_call_select=Generate Function Call Signal  TaskName='Task1'  Poll_timeout=-1  Ts=SamTime
      settings: SourceProductName=Pixhawk Target Blocks
  wires:
  CmdGenerator/5(isSendCmd) -> vehicle_commander/9
  CmdGenerator/1(cmd) -> Data Type Conversion/1
  isEnCtrl/1 -> CmdGenerator/1(isEnCtrl)
  CmdGenerator/7(isSendBlock) -> RePX4Block/1
  Bus Selector/1 -> vehicle_commander/7, vehicle_commander/5  "<system_id>"
  CmdGenerator/3(params2) -> vehicle_commander/2
  Bus Selector/2 -> vehicle_commander/8, vehicle_commander/6  "<component_id>"
  CmdGenerator/2(params1) -> vehicle_commander/1
  CmdGenerator/8(blockmode) -> RePX4Block/2
  CmdGenerator/4(params3) -> vehicle_commander/3
  AutoBlock/1 -> CmdGenerator/5(isAutoBlock)
  AutoLoiter/1 -> CmdGenerator/6(isAutoLoiter)
  AutoArm/1 -> CmdGenerator/4(isAutoArm)
  Clock/1 -> CmdGenerator/2(t)
  vehicle_status/1 -> Bus Selector/1
  Mode/1 -> CmdGenerator/3(mode)
  MATLAB Function1/1(y) -> Demux/1
  Constant/1 -> MATLAB Function1/2(idxList)
  Ctrls/1 -> MATLAB Function1/1(u)
  CmdGenerator/6(isSendOff) -> uORB Write Advanced_dai1/13
  Data Type Conversion/1 -> vehicle_commander/4
  Sum/1 -> uORB Write Advanced_dai1/4
  Constant3/1 -> Sum/2
  Gain/1 -> Sum/1
  Demux/4 -> Gain/1
  Constant2/1 -> uORB Write Advanced_dai1/1
  Demux/1 -> uORB Write Advanced_dai1/3
  Demux/2 -> uORB Write Advanced_dai1/2
  Demux/3 -> uORB Write Advanced_dai1/5
  Demux/5 -> uORB Write Advanced_dai1/6
  Demux/6 -> uORB Write Advanced_dai1/7
  Demux/7 -> uORB Write Advanced_dai1/8
  Demux/8 -> uORB Write Advanced_dai1/9
  Demux/9 -> uORB Write Advanced_dai1/10
  Demux/10 -> uORB Write Advanced_dai1/11
  Demux/11 -> uORB Write Advanced_dai1/12

== system pixhawk_slib_rfly/RePX4Block ==
  note: mode
      | 0: 不屏蔽PX4输出，使用PX4官方控制器，不接收平台IO和Sim控制量。这个模式需要配合Offboard接口（包括：HIL16Ctrls、OffboardPvaCtrlAPI、OffboardAdvCtrlAPI、OffboardAttCtrlAPI、HIL16CtrlsNorm等）
      | 1：屏蔽PX4输出。会同时屏蔽力矩层、IO层和仿真层消息的输出。
      | 2：只屏蔽PX4的力矩层，需要Simulink发送力和力矩信号（配合使用TorqueThrustCtrls接口）控制飞机。这种模式适用于所有电调格式（PWM或DSHOT等）、所有飞机输出。
  note: bool armed		// 这个表示是否切换到RflySim的HIL_output硬件在环仿真输出.
      | 注：设置为true，表示仿真器会接收rfly硬件在环仿真消息actuator_outputs_rlfy，而不是官方消息actuator_outputs
      | 也就是说，本质上控制了是响应PX4的硬件在环控制量还是Simulink的硬件在环仿真控制量。
      | 设置为false，接收PX4官方仿真actuator_outputs消息，能够正常用遥控器完成全功能。
      |
      | bool prearmed //这个表示是否切换到RflySim的actuator_controls_0消息。
      | 注：设置为true，接收RflySim的力和力矩控制信号actuator_controls_rfly（1.13及之前）或vehicle_torque/thrust_setpoint_rfly（1.14及之后）
      | 设置为false，使用PX4官网控制信号actuator_controls_0（1.13及之前）或vehicle_torque/thrust_setpoint0（1.14及之后）
      |
      |
      | bool ready_to_arm //这个表示，切换到Rfly的电机/舵机真机输出。
      | 注：设置为true，会屏蔽PX4底层对电机的访问，无法控制电机。只能用平台PWM_output 和 Aux_output接口控制。
      | 设置为false，会屏蔽RflySim的PWM_output 和 Aux_output接口控制接口，开发PX4官方控制器。
  note: armed: simulation switch: true for rfly HILSim ctrls (actuator_outputs_rlfy) or false for px4 sim ctrls (actuator_outputs)
      | prearmed: actuator_controls_0 (torque and thrust control) block flag: true for blocking PX4 torque and thrust ctrls
      | ready_to_arm: motor and servo block flag: true to block px4 output.
  isEnCtrl : Inport  OutDataTypeStr=boolean
  mode : Inport  Port=2  OutDataTypeStr=uint8  PortDimensions=1
  ModeSwitch : MATLAB Function  TreatAsAtomicUnit=on  SystemSampleTime=SamTime
  actuator_armed_rfly : pixhawk_slib_uORB_RW/uORB Write Advanced_dai  Ts=0  uORB_AdvtQueue=on  uORB_FieldEnabledArr="0  0  0  1  0  0  0  0  0  0  0"  uORB_Topic_str=0  uORB_Topic_str_ID=0  uORB_Struct_DT="[1  1  1  1  1]"  BlockInputCount=5  uORB_StructParams="[\"voltage_v\",\"voltage_filtered_v\",\"current_a\",\"current_filtered_a\",\"remaining\"]"  uORB_PortSizes="[1  1  1  1]"  MsgSizeOf=0  MW_update=true
      settings: SourceProductName=Pixhawk Target Blocks
  wires:
  ModeSwitch/1(isSim) -> actuator_armed_rfly/1
  ModeSwitch/3(isIO) -> actuator_armed_rfly/3
  mode/1 -> ModeSwitch/2(dState)
  ModeSwitch/2(isTor) -> actuator_armed_rfly/2
  ModeSwitch/5(isSend) -> actuator_armed_rfly/5
  isEnCtrl/1 -> ModeSwitch/1(isEn)
  ModeSwitch/4(isRC) -> actuator_armed_rfly/4

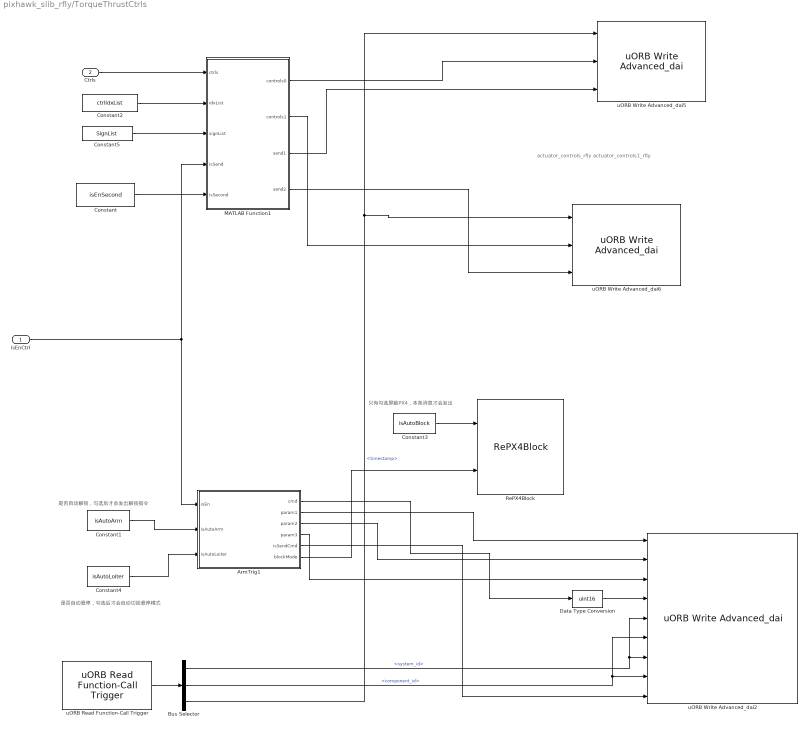
== system pixhawk_slib_rfly/TorqueThrustCtrls ==
  note: actuator_controls_rfly actuator_controls1_rfly
  note: 只有勾选屏蔽PX4，本条消息才会发出
  note: 是否自动悬停，勾选后才会自动切回悬停模式
  note: 是否自动解锁，勾选后才会发出解锁指令
  isEnCtrl : Inport  OutDataTypeStr=boolean
  Ctrls : Inport  Port=2  OutDataTypeStr=single  PortDimensions=4
  ArmTrig1 : MATLAB Function  TreatAsAtomicUnit=on  SystemSampleTime=SamTime
  Bus Selector : BusSelector  OutputSignals=system_id,component_id,timestamp
  Constant : Constant  Value=isEnSecond  OutDataTypeStr=boolean
  Constant1 : Constant  Value=isAutoArm  OutDataTypeStr=boolean
  Constant2 : Constant  Value=ctrlIdxList
  Constant3 : Constant  Value=isAutoBlock  OutDataTypeStr=boolean
  Constant4 : Constant  Value=isAutoLoiter  OutDataTypeStr=boolean
  Constant5 : Constant  Value=SignList
  Data Type Conversion : DataTypeConversion  OutDataTypeStr=uint16  SaturateOnIntegerOverflow=off  RndMeth=Floor
  MATLAB Function1 : MATLAB Function  TreatAsAtomicUnit=on  SystemSampleTime=SamTime
  RePX4Block : $bdroot/RePX4Block  SamTime=SamTime
  uORB Read Function-Call Trigger : pixhawk_slib_uORB_RW/uORB Read Function-Call Trigger  uORB_Topic_str='vehicle_status'  BusObjVar=Bus: vehicle_status_SL  uORB_Interval=4  AsyncOutput=off  Fcn_call_select=Generate Function Call Signal  TaskName='Task1'  Poll_timeout=-1  Ts=SamTime
      settings: SourceProductName=Pixhawk Target Blocks
  uORB Write Advanced_dai2 : pixhawk_slib_uORB_RW/uORB Write Advanced_dai  Ts=0  uORB_AdvtQueue=on  uORB_FieldEnabledArr="0  0  0  1  0  0  0  0  0  0  0"  uORB_Topic_str=0  uORB_Topic_str_ID=0  uORB_Struct_DT="[1  1  1  1  1]"  BlockInputCount=5  uORB_StructParams="[\"voltage_v\",\"voltage_filtered_v\",\"current_a\",\"current_filtered_a\",\"remaining\"]"  uORB_PortSizes="[1  1  1  1]"  MsgSizeOf=0  MW_update=true
      settings: SourceProductName=Pixhawk Target Blocks
  uORB Write Advanced_dai5 : pixhawk_slib_uORB_RW/uORB Write Advanced_dai  Ts=0  uORB_AdvtQueue=on  uORB_FieldEnabledArr="0  0  0  1  0  0  0  0  0  0  0"  uORB_Topic_str=0  uORB_Topic_str_ID=0  uORB_Struct_DT="[1  1  1  1  1]"  BlockInputCount=5  uORB_StructParams="[\"voltage_v\",\"voltage_filtered_v\",\"current_a\",\"current_filtered_a\",\"remaining\"]"  uORB_PortSizes="[1  1  1  1]"  MsgSizeOf=0  MW_update=true
      settings: SourceProductName=Pixhawk Target Blocks
  uORB Write Advanced_dai6 : pixhawk_slib_uORB_RW/uORB Write Advanced_dai  Ts=0  uORB_AdvtQueue=on  uORB_FieldEnabledArr="0  0  0  1  0  0  0  0  0  0  0"  uORB_Topic_str=0  uORB_Topic_str_ID=0  uORB_Struct_DT="[1  1  1  1  1]"  BlockInputCount=5  uORB_StructParams="[\"voltage_v\",\"voltage_filtered_v\",\"current_a\",\"current_filtered_a\",\"remaining\"]"  uORB_PortSizes="[1  1  1  1]"  MsgSizeOf=0  MW_update=true
      settings: SourceProductName=Pixhawk Target Blocks
  wires:
  Constant2/1 -> MATLAB Function1/2(idxList)
  Ctrls/1 -> MATLAB Function1/1(ctrls)
  MATLAB Function1/4(send2) -> uORB Write Advanced_dai6/3
  Constant5/1 -> MATLAB Function1/3(signList)
  Constant/1 -> MATLAB Function1/5(isSecond)
  MATLAB Function1/3(send1) -> uORB Write Advanced_dai5/3
  ArmTrig1/6(blockMode) -> RePX4Block/2
  ArmTrig1/1(cmd) -> Data Type Conversion/1
  Bus Selector/2 -> uORB Write Advanced_dai2/8, uORB Write Advanced_dai2/6  "<component_id>"
  ArmTrig1/5(isSendCmd) -> uORB Write Advanced_dai2/9
  ArmTrig1/3(param2) -> uORB Write Advanced_dai2/2
  ArmTrig1/4(param3) -> uORB Write Advanced_dai2/3
  Bus Selector/1 -> uORB Write Advanced_dai2/5, uORB Write Advanced_dai2/7  "<system_id>"
  ArmTrig1/2(param1) -> uORB Write Advanced_dai2/1
  Constant3/1 -> RePX4Block/1
  uORB Read Function-Call Trigger/1 -> Bus Selector/1
  Constant4/1 -> ArmTrig1/3(isAutoLoiter)
  Constant1/1 -> ArmTrig1/2(isAutoArm)
  isEnCtrl/1 -> ArmTrig1/1(isEn), MATLAB Function1/4(isSend)
  Bus Selector/3 -> uORB Write Advanced_dai6/1, uORB Write Advanced_dai5/1  "<timestamp>"
  MATLAB Function1/2(controls1) -> uORB Write Advanced_dai6/2
  MATLAB Function1/1(controls0) -> uORB Write Advanced_dai5/2
  Data Type Conversion/1 -> uORB Write Advanced_dai2/4

== matlab function pixhawk_slib_rfly/OffboardAttCtrlAPI/SwitchForVtol ==
  data: isSend input; isSendAtt output; isSendAttMc output; isSendAttFw output; isSendRate output; is_vtol input; vehicle_type input; isAttMode input; isRateMode input
function [isSendAtt,isSendAttMc,isSendAttFw,isSendRate] = fcn(isSend,is_vtol,vehicle_type,isAttMode,isRateMode)
isSendAtt=0;
isSendAttMc=0;
isSendAttFw=0;
isSendRate=0;

if isSend>0.5
    if isAttMode
        if is_vtol && vehicle_type==1 %VEHICLE_TYPE_ROTARY_WING = 1;
            isSendAttMc=1;
        elseif is_vtol && vehicle_type==2 %VEHICLE_TYPE_FIXED_WING = 2;
            isSendAttFw=1;
        else
            isSendAtt=1;
        end
    else
        if isRateMode
            isSendRate=1;
        end
    end
end

== matlab function pixhawk_slib_rfly/OffboardAttCtrlAPI/AttCtrlMap ==
  data: Ctrls input; MapList input; AttEuler3d output; AttQuat4d output; AttRate3d output; Thrust3d output; isEnList input; isAttMode output; isRateMode output
function [AttEuler3d,AttQuat4d,AttRate3d,Thrust3d,isAttMode,isRateMode] = fcn(Ctrls,MapList,isEnList)

tVect=single(NaN(13,1));

for i=1:length(Ctrls)
    tVect(MapList(i))=Ctrls(i);
end

AttEuler3d=tVect(1:3);
AttQuat4d=tVect(4:7);
AttRate3d=tVect(8:10);
Thrust3d=tVect(11:13);

isEuler=isEnList(1);
isQuat=isEnList(2);
isRollR=isEnList(3);
isPitchR=isEnList(4);
isYawR=isEnList(5);

isAttMode=false;

if isEuler || isQuat
    isAttMode=true;
    
    if isEuler
        roll=AttEuler3d(1);
        pitch=AttEuler3d(2);
        yaw=AttEuler3d(3);
        sp2=sin(pitch/2);
        sy2=sin(yaw/2);
        cr2=cos(roll/2);
        cp2=cos(pitch/2);
        cy2=cos(yaw/2);
        sr2=sin(roll/2);

        qx=sp2*sy2*cr2+cp2*cy2*sr2;
        qy=sp2*cy2*cr2+cp2*sy2*sr2;
        qz=cp2*sy2*cr2-sp2*cy2*sr2;
        qw=cp2*cy2*cr2-sp2*sy2*sr2;
        AttQuat4d=[qw;qx;qy;qz];
        
    end
    if isQuat
        %AttEuler3d=quat2eul(AttQuat4d);
        
        % Normalize the quaternions 归一化四元数
        norm_q = sqrt(sum(AttQuat4d.^2));
        AttQuat4d = AttQuat4d ./ norm_q;

        if (AttQuat4d(1)<0) % 如果标量为负号，则乘以-1
            AttQuat4d=-AttQuat4d;
        end
    
        % Quat to Euler
        qw = AttQuat4d(1);
        qx = AttQuat4d(2);
        qy = AttQuat4d(3);
        qz = AttQuat4d(4);
        % under some circumstances.
        AttEuler3d=[ atan2( 2*(qx.*qy+qw.*qz), qw.^2 + qx.^2 - qy.^2 - qz.^2 ); ...
            asin( -2*(qx.*qz-qw.*qy) ); ...
            atan2( 2*(qy.*qz+qw.*qx), qw.^2 - qx.^2 - qy.^2 + qz.^2 )];
    end
    
end

isRateMode=false;
if isRollR || isPitchR || isYawR
    isRateMode=true;
    if ~isRollR && ~isPitchR && isAttMode
        isRateMode=false;
    end
end

== matlab function pixhawk_slib_rfly/RCOverCtrlAPI/CmdGenerator ==
  data: isEnCtrl input; cmd output; params1 output; params2 output; params3 output; isSendCmd output; t input; mode input; isSendOff output; isAutoArm input; isAutoBlock input; isSendBlock output; isAutoLoiter input; blockmode output
function [cmd,params1,params2,params3,isSendCmd,isSendOff,isSendBlock,blockmode] = fcn(isEnCtrl,t,mode,isAutoArm,isAutoBlock,isAutoLoiter)


persistent lastT;
persistent flag;
persistent lastEnCtrl;

isSendBlock=false;
blockmode=uint8(0);
if isempty(lastT)
    lastT=0;
end

if isempty(flag)
    flag=0;
end



if isempty(lastEnCtrl)
    lastEnCtrl=false;
    if isAutoBlock
        isSendBlock=true;
    end
end

isSendCmd=0;
isSendOff=0;

cmd=uint32(0);
params1=single(NaN);
params2=single(NaN);
params3=single(NaN);



if lastEnCtrl~= isEnCtrl% 不相等
    lastEnCtrl = isEnCtrl;
    
    if isAutoBlock
        isSendBlock=true;
    end
    
    
    if isEnCtrl % 使能Offboard
        blockmode=uint8(3); % 屏蔽RC的模式
        if isAutoArm
            flag=1; % 进入等待Offboard模式切换指令   
            
            isSendCmd=1; % 发送命令
            cmd=uint32(400); %MAV_CMD_COMPONENT_ARM_DISARM
            params1=single(1); %  Arm
            params2=single(0); %  No Force
            
        else
            flag=2; % 直接进入发送数据模式
        end

%         % 切换指定模式
%         isSendCmd=1; % 发送命令
%         cmd=uint32(176); %MAV_CMD_DO_SET_MODE
%         params1=single(1); % Mode
%         params2=single(mode); % Custom Mode: PX4_CUSTOM_MAIN_MODE_OFFBOARD
        
        
    else % 禁用Offboard
        
        flag=0;
        if isAutoLoiter % 如果启用自动悬停，就进入悬停模式
            isSendCmd=1; % 发送命令
            cmd=uint32(176); %MAV_CMD_DO_SET_MODE
            params1=single(1); % Mode
            params2=single(4); % Custom Mode: PX4_CUSTOM_MAIN_MODE_AUTO
            params3=single(3); % Custom Submode: PX4_CUSTOM_SUB_MODE_AUTO_LOITER
            % 切换到定点模式
        end

    end
    
    lastT=t;
end

if abs(flag-1)<0.01 && (t-lastT)>0.5 % 发送offboard数据0.5秒收
    flag=2;
    isSendCmd=1; % 发送命令
    cmd=uint32(176); %MAV_CMD_DO_SET_MODE
    params1=single(1); % Mode
    params2=single(mode); % Custom Mode: PX4_CUSTOM_MAIN_MODE_OFFBOARD
end



% 只要在Offboard发送模式，就发送Offboard消息
if flag>1.5 && flag<3.5
    isSendOff=1; % 开始发送Offboard消息 % 解锁完成后，才发送遥控器数据。避免高油门解锁失败。
    
end

== matlab function pixhawk_slib_rfly/RCOverCtrlAPI/MATLAB Function1 ==
  data: u input; y output; idxList input
function y = fcn(u,idxList)
y=single(NaN(11,1));
for i=1:length(u)
    y(idxList(i))=u(i);
end

== matlab function pixhawk_slib_rfly/TorqueThrustCtrls/MATLAB Function1 ==
  data: ctrls input; controls0 output size=8; controls1 output size=8; idxList input; signList input; isSend input; isSecond input; send1 output; send2 output
function [controls0,controls1,send1,send2] = fcn(ctrls,idxList,signList,isSend,isSecond)

% MAV_TYPE_GROUND_ROVER=10,thrust_body_array[0] = thrust;
% MAV_TYPE_FIXED_WING=1 同上
%MAV_TYPE_SUBMARINE=12, /* Submarine | */

CtrlsAll=single(zeros(12,1));
send1=0;
send2=0;
if isSend
    for i=1:length(ctrls)
        CtrlsAll(idxList(i))=ctrls(i)*signList(i);
    end
    send1=1;
    if isSecond
        send2=1;
    end
end

torque=CtrlsAll(1:3,:);
thrust=CtrlsAll(4:6,:);
torque1=CtrlsAll(7:9,:);
thrust1=CtrlsAll(10:12,:);

 controls0=[torque;-thrust(3);0;0;0;0;];
 controls1=[torque1;-thrust1(3);0;0;0;0;];

== matlab function pixhawk_slib_rfly/OffboardAdvCtrlAPI/OffboardManage ==
  data: PVAYR input; Pxyz output; EnList input; Vxyz output; Axyz output; yaw output; yawRate output; isPos output; isVel output; isAcc output
function [Pxyz,Vxyz,Axyz,yaw,yawRate,isPos,isVel,isAcc] = fcn(PVAYR,EnList)

PVAYR_out=single(NaN(11,1));

isPos=false;
isVel=false;
isAcc=false;

for i=1:length(EnList)
    if EnList(i)
        PVAYR_out(i)=PVAYR(i);
    end
end

Pxyz=PVAYR_out(1:3);
Vxyz=PVAYR_out(4:6);
Axyz=PVAYR_out(7:9);
yaw=PVAYR_out(10);
yawRate=PVAYR_out(11);


if EnList(1) || EnList(2) || EnList(3) % 勾选启用位置控制项
    if ~isnan(Pxyz(1)) || ~isnan(Pxyz(2)) || ~isnan(Pxyz(3))  % 且不全为NaN
        isPos=true;
    end
end
if EnList(4) || EnList(5) || EnList(6)  % 勾选启用速度控制项
    if ~isnan(Vxyz(1)) || ~isnan(Vxyz(2)) || ~isnan(Vxyz(3))  % 且不全为NaN
        isVel=true;
    end
end
if EnList(7) || EnList(8) || EnList(9) % 勾选启用加速度控制项
    if ~isnan(Axyz(1)) || ~isnan(Axyz(2)) || ~isnan(Axyz(3))  % 且不全为NaN
        isAcc=true;
    end
end

== matlab function pixhawk_slib_rfly/RePX4Block/ModeSwitch ==
  data: isEn input; dState input; isSim output; isTor output; isIO output; isRC output; isSend output
function [isSim,isTor,isIO,isRC,isSend] = fcn(isEn,dState)

isSend=0;
persistent lastState;
persistent lastEn;
if isempty(lastState)
    lastState=uint8(0);
    if isEn
        isSend=1;
    end
end

if isempty(lastEn)
    lastEn=false;
end

% 默认不屏蔽输出
isSim=false;
isTor=false;
isIO=false;
isRC=false;

if dState~=lastState || isEn~=lastEn % 两种情况都会触发消息发送
    lastState=dState;
    lastEn=isEn;
    if dState>2.5 % 只屏蔽controls0的力和力矩输出
        isRC=true;
        isSim=false;
        isTor=false;
        isIO=false;
    elseif dState>1.5 % 只屏蔽controls0的力和力矩输出
        isSim=false;
        isTor=true;
        isIO=false;

    elseif dState>0.5 % 屏蔽PX4的所有输出
        isSim=true;
        isTor=false;
        isIO=true;
    end
    
    if isEn
        isSend=1;
    end

end

== matlab function pixhawk_slib_rfly/HIL16CtrlsPWM/ArmTrig1 ==
  data: isEn input; cmd output; param1 output; param2 output; param3 output; isSendCmd output; isAutoArm input; isAutoLoiter input; blockMode output
function [cmd,param1,param2,param3,isSendCmd,blockMode] = fcn(isEn,isAutoArm,isAutoLoiter)

persistent lastEnState;
if isempty(lastEnState)
    lastEnState=false;
end


cmd=uint32(0); % 默认空指令
param1=single(0);
param2=single(0);
param3=single(0);
isSendCmd=0; % 不发送

if isEn % 使能的话，就要屏蔽输出
    blockMode=uint8(1); % 如果置于1，则屏蔽输出
else
    blockMode=uint8(0); % 默认不屏蔽输出
end

if isEn~=lastEnState % 不相等，就会触发本循环
    lastEnState=isEn;
    
    if isEn && isAutoArm % 如果开启自动解锁，就解锁飞控
        isSendCmd=1; % 本轮发送
        cmd=uint32(400); %MAV_CMD_COMPONENT_ARM_DISARM，解锁或上锁指令
        param1=single(1); %  Arm 解锁
        param2=single(0); %  No Force 不强制
    end
    
    if ~isEn && isAutoLoiter % 如果开启自动解锁，就解锁飞控
        isSendCmd=1; % 本轮发送
        cmd=uint32(176); %MAV_CMD_DO_SET_MODE 模式设置指令
        param1=single(1); % Mode 设为1，表示确认设置
        param2=single(4); % Custom Mode: PX4_CUSTOM_MAIN_MODE_AUTO 自动模式
        param3=single(3); % Custom Submode: PX4_CUSTOM_SUB_MODE_AUTO_LOITER 悬停子模式
        % 切换到定点模式
        
    end

    
end

== matlab function pixhawk_slib_rfly/OffboardPvaCtrlAPI/MATLAB Function1 ==
  data: u input; ignore_thrust output; ignore_attitude output; ignore_bodyrate_x output; ignore_bodyrate_y output; ignore_bodyrate_z output; ignore_position output; ignore_velocity output; ignore_acceleration_force output; ignore_alt_hold output
function [ignore_thrust,ignore_attitude,ignore_bodyrate_x,ignore_bodyrate_y,ignore_bodyrate_z,ignore_position,ignore_velocity,ignore_acceleration_force,ignore_alt_hold] = fcn(u)


isX=u(1);
isY=u(2);
isZ=u(3);
isVx=u(4);
isVy=u(5);
isVz=u(6);
isAx=u(7);
isAy=u(8);
isAz=u(9);
isYaw=u(10);
isYawRate=u(11);


ignore_thrust=true;
ignore_attitude=true;
ignore_bodyrate_x=true;
ignore_bodyrate_y=true;
ignore_bodyrate_z=true;

ignore_position=false;
ignore_velocity=false;
ignore_acceleration_force=false;
ignore_alt_hold=false;

if ~isX && ~isY && ~isZ
    ignore_position=true;
end

if ~isVx && ~isVy && ~isVz
    ignore_velocity=true;
end

if ~isAx && ~isAy && ~isAz
    ignore_acceleration_force=true;
end

if isYaw % 有偏航角，就不禁用
    ignore_attitude=false;
end

if isYawRate % 有偏航角速度，就不禁用
    ignore_bodyrate_z=false;
end

if isVz
    ignore_alt_hold=true;
end

== matlab function pixhawk_slib_rfly/HIL16CtrlsNorm/ArmTrig1 ==
  data: isEn input; cmd output; param1 output; param2 output; param3 output; isSendCmd output; isAutoArm input; isAutoLoiter input; blockMode output
function [cmd,param1,param2,param3,isSendCmd,blockMode] = fcn(isEn,isAutoArm,isAutoLoiter)

persistent lastEnState;
if isempty(lastEnState)
    lastEnState=false;
end


cmd=uint32(0); % 默认空指令
param1=single(0);
param2=single(0);
param3=single(0);
isSendCmd=0; % 不发送

if isEn % 使能的话，就要屏蔽输出
    blockMode=uint8(1); % 如果置于1，则屏蔽输出
else
    blockMode=uint8(0); % 默认不屏蔽输出
end

if isEn~=lastEnState % 不相等，就会触发本循环
    lastEnState=isEn;
    
    if isEn && isAutoArm % 如果开启自动解锁，就解锁飞控
        isSendCmd=1; % 本轮发送
        cmd=uint32(400); %MAV_CMD_COMPONENT_ARM_DISARM，解锁或上锁指令
        param1=single(1); %  Arm 解锁
        param2=single(0); %  No Force 不强制
    end
    
    if ~isEn && isAutoLoiter % 如果开启自动解锁，就解锁飞控
        isSendCmd=1; % 本轮发送
        cmd=uint32(176); %MAV_CMD_DO_SET_MODE 模式设置指令
        param1=single(1); % Mode 设为1，表示确认设置
        param2=single(4); % Custom Mode: PX4_CUSTOM_MAIN_MODE_AUTO 自动模式
        param3=single(3); % Custom Submode: PX4_CUSTOM_SUB_MODE_AUTO_LOITER 悬停子模式
        % 切换到定点模式
        
    end

    
end

== matlab function pixhawk_slib_rfly/OffboardPvaCtrlAPI/OffboardManage ==
  data: PVAYR input; Pxyz output; EnList input; Vxyz output; Axyz output; yaw output; yawRate output; isPos output; isVel output; isAcc output
function [Pxyz,Vxyz,Axyz,yaw,yawRate,isPos,isVel,isAcc] = fcn(PVAYR,EnList)

PVAYR_out=single(NaN(11,1));

isPos=false;
isVel=false;
isAcc=false;

for i=1:length(EnList)
    if EnList(i)
        PVAYR_out(i)=PVAYR(i);
    end
end

Pxyz=PVAYR_out(1:3);
Vxyz=PVAYR_out(4:6);
Axyz=PVAYR_out(7:9);
yaw=PVAYR_out(10);
yawRate=PVAYR_out(11);


if EnList(1) || EnList(2) || EnList(3) % 勾选启用位置控制项
    if ~isnan(Pxyz(1)) || ~isnan(Pxyz(2)) || ~isnan(Pxyz(3))  % 且不全为NaN
        isPos=true;
    end
end
if EnList(4) || EnList(5) || EnList(6)  % 勾选启用速度控制项
    if ~isnan(Vxyz(1)) || ~isnan(Vxyz(2)) || ~isnan(Vxyz(3))  % 且不全为NaN
        isVel=true;
    end
end
if EnList(7) || EnList(8) || EnList(9) % 勾选启用加速度控制项
    if ~isnan(Axyz(1)) || ~isnan(Axyz(2)) || ~isnan(Axyz(3))  % 且不全为NaN
        isAcc=true;
    end
end

== matlab function pixhawk_slib_rfly/OffboardAttCtrlAPI/MATLAB Function3 ==
  data: u input; ignore_thrust output; ignore_attitude output; ignore_bodyrate_x output; ignore_bodyrate_y output; ignore_bodyrate_z output; ignore_position output; ignore_velocity output; ignore_acceleration_force output; ignore_alt_hold output
function [ignore_thrust,ignore_attitude,ignore_bodyrate_x,ignore_bodyrate_y,ignore_bodyrate_z,ignore_position,ignore_velocity,ignore_acceleration_force,ignore_alt_hold] = fcn(u)

isEuler=u(1);
isQuat=u(2);
isRollR=u(3);
isPitchR=u(4);
isYawR=u(5);
isThrust=u(6);

ignore_thrust=false;
ignore_attitude=false;
ignore_bodyrate_x=false;
ignore_bodyrate_y=false;
ignore_bodyrate_z=false;

ignore_position=true;
ignore_velocity=true;
ignore_acceleration_force=true;
ignore_alt_hold=true;


if ~isEuler && ~isQuat
    ignore_attitude=true;
end

if ~isRollR
    ignore_bodyrate_x=true;
end

if ~isPitchR
    ignore_bodyrate_y=true;
end

if ~isYawR
    ignore_bodyrate_z=true;
end


if ~isThrust
    ignore_thrust=true;
end

== matlab function pixhawk_slib_rfly/OffboardAttCtrlAPI/MATLAB Function ==
  data: isVtol input; vehicle_type output; isRoWing input
function vehicle_type = fcn(isVtol,isRoWing)

if isVtol
    if isRoWing
        vehicle_type=uint8(1);
    else
        vehicle_type=uint8(2);
    end 
else
    vehicle_type=uint8(0);
end

== matlab function pixhawk_slib_rfly/OffCtrlMsgAll/MATLAB Function ==
  data: position output; ignore_attitude input; ignore_bodyrate input; ignore_position input; ignore_velocity input; ignore_acceleration_force input; velocity output; acceleration output; attitude output; body_rate output
function [position,velocity,acceleration,attitude,body_rate] = fcn(ignore_attitude,ignore_bodyrate,ignore_position,ignore_velocity,ignore_acceleration_force)
% bool position
% bool velocity
% bool acceleration
% bool attitude
% bool body_rate
% bool actuator

% bool ignore_thrust
% bool ignore_attitude
% bool ignore_bodyrate
% bool ignore_position
% bool ignore_velocity
% bool ignore_acceleration_force
% bool ignore_alt_hold

position=~ignore_position;
velocity=~ignore_velocity;
acceleration=~ignore_acceleration_force;
attitude=~ignore_attitude;
body_rate=~ignore_bodyrate;
